simulink library "HORTISIM"  (R2021a)
settings: Solver=VariableStepAuto  StartTime=0.0  StopTime=10.0  RelTol=1e-3
undefined symbols (not defined in the file or in its folder): crop_params, heat_ic, heat_p, p_climate, params_fruit, scr_p, substrate_params, tp_tilapia, win_p, x0_climate, x0_crop, x0_fruit, x0_substrate, x0_tank_tilapia
libraries: $bdroot x10
(part 1 of 4)
settings Model: Creator=djoroya  LastModifiedBy=djoroya

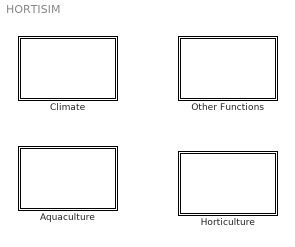
== system HORTISIM ==
  Aquaculture : Subsystem
  Climate : Subsystem
  Horticulture : Subsystem
  Other Functions : Subsystem

== system HORTISIM/Aquaculture ==
  Controls : Subsystem
  Models : Subsystem

== system HORTISIM/Climate ==
  Controls : Subsystem
  Models : Subsystem

== system HORTISIM/Horticulture ==
  Controls : Subsystem
  Models : Subsystem

== system HORTISIM/Other Functions ==
  Scalar2Bus Control Crop : Subsystem
  Scalar2Bus Control Climate : Subsystem
  Screen Connector : Subsystem
  Sec2Days : Gain  Gain=24*3600
  Temp2SatDensity : Subsystem
  Windows Connector : Subsystem
  Zero Element Screen : Subsystem
  Zero Element Windows : Subsystem
  cumfun : Subsystem
  parseExteriorClima : Subsystem
  sigmoi : Subsystem  mask{sigma=0}

== system HORTISIM/Aquaculture/Controls ==

== system HORTISIM/Aquaculture/Models ==
  Filter Species : Subsystem
      mask Display: image('$imagefile'); % Use "Edit Image" on toolstrip to change.
  Tank Model : Subsystem  mask{x0=x0_tank_tilapia, params=tp_tilapia}
      settings: PortSchema="{\"entries\":[{\"content\":{\"sides\":[{\"content\":{\"connectorIds\":[\"In1\",\"In2\"]},\"type\":\"ConnectorPlacement.EquallySpacedRectSide\",\"uuid\":\"0362ec3b-d1e8-482f-a4df-c7eb6405d3bb\"},{\"content\":{\"connectorIds\":[\"Out1\"],\"side\":\"RIGHT\"},\"type\":\"ConnectorPlacement.EquallySpacedRectSide\",\"uuid\":\"883d7bea-5680-4a36-94aa-1bdc656ec6e4\"},{\"content\":{\"connectorIds\":[\"In3\"],\"side\":\"TOP\"},\"type\":\"ConnectorPlacement.EquallySpacedRectSide\",\"uuid\":\"cb609290-e3df-4833-81b0-31186814fdae\"},{\"content\":{\"connectorIds\":[\"In4\",\"In5\"],\"side\":\"BOTTOM\"},\"type\":\"ConnectorPlacement.EquallySpacedRectSide\",\"uuid\":\"90a50527-453f-4e54-bcbc-22902a66f901\"}]},\"type\":\"ConnectorPlacement.EquallySpacedConnector\",\"uuid\":\"8e8832ba-26f8-49e0-87fc-105394dbe278\"}],\"packageUris\":[\"http://schema.mathworks.com/mf0/Connector/R2020b\"],\"version\":\"1.0\"}"
      mask Display: image('$imagefile'); % Use "Edit Image" on toolstrip to change.

== system HORTISIM/Climate/Controls ==
  CO2 Pump : Subsystem
      mask Display: image('$imagefile'); % Use "Edit Image" on toolstrip to change.
  Fogging Controler : Subsystem
      mask Display: image('$imagefile'); % Use "Edit Image" on toolstrip to change.
  Heating Controler : Subsystem  mask{params=heat_p, x0=heat_ic}
      mask Display: image('$imagefile'); % Use "Edit Image" on toolstrip to change.
  Screen Controler : Subsystem  mask{params=scr_p}
      mask Display: image('$imagefile'); % Use "Edit Image" on toolstrip to change.
  Windows Controler : Subsystem  mask{params=win_p}
      mask Display: image('$imagefile'); % Use "Edit Image" on toolstrip to change.

== system HORTISIM/Climate/Models ==
  Climate Model : Subsystem  mask{params=p_climate, x0=x0_climate}
      mask Display: image('$imagefile'); % Use "Edit Image" on toolstrip to change.

== system HORTISIM/Horticulture/Controls ==
  Ferrtirrigation Controler : Subsystem
      mask Display: image('$imagefile'); % Use "Edit Image" on toolstrip to change.
  Prune Policy : Subsystem
      mask Display: image('$imagefile'); % Use "Edit Image" on toolstrip to change.

== system HORTISIM/Horticulture/Models ==
  Crop Grow : Subsystem  mask{params=crop_params, x0=x0_crop}
      settings: PortSchema="{\"entries\":[{\"content\":{\"sides\":[{\"content\":{\"connectorIds\":[\"In1\"]},\"type\":\"ConnectorPlacement.EquallySpacedRectSide\",\"uuid\":\"7d52d4c6-bc72-40ae-ba7a-fef791f60555\"},{\"content\":{\"connectorIds\":[\"Out1\"],\"side\":\"RIGHT\"},\"type\":\"ConnectorPlacement.EquallySpacedRectSide\",\"uuid\":\"3a9c2840-361d-4677-a7cc-c5f954b33f07\"},{\"content\":{\"connectorIds\":[\"In2\",\"In3\"],\"side\":\"TOP\"},\"type\":\"ConnectorPlacement.EquallySpacedRectSide\",\"uuid\":\"4fc8b0ee-86a8-4f1e-9fcc-25f95949aa32\"},{\"content\":{\"connectorIds\":[],\"side\":\"BOTTOM\"},\"type\":\"ConnectorPlacement.EquallySpacedRectSide\",\"uuid\":\"254dc665-acaf-49d5-9184-a028de083de6\"}]},\"type\":\"ConnectorPlacement.EquallySpacedConnector\",\"uuid\":\"4a2a8912-594b-41a4-9c04-2b6ae0329b55\"}],\"packageUris\":[\"http://schema.mathworks.com/mf0/Connector/R2020b\"],\"version\":\"1.0\"}"
      mask Display: image('$imagefile'); % Use "Edit Image" on toolstrip to change.
  Fruit Partitioning1 : Subsystem  mask{x0=x0_fruit, params=params_fruit}
      mask Display: image('$imagefile'); % Use "Edit Image" on toolstrip to change.
  Substrate Bag : Subsystem  mask{x0=x0_substrate, params=substrate_params}
      mask Display: image('$imagefile'); % Use "Edit Image" on toolstrip to change.

== system HORTISIM/Other Functions/Scalar2Bus Control Crop ==
  Prune : Inport
  Harvest : Inport  Port=2
  Artificial Rad : Inport  Port=3
  Bus Creator : BusCreator  Inputs=3
  out : Outport
  wires:
  Prune/1 -> Bus Creator/1  "Prune"
  Harvest/1 -> Bus Creator/2  "Harvest"
  Artificial Rad/1 -> Bus Creator/3  "Artificial Rad"
  Bus Creator/1 -> out/1

== system HORTISIM/Other Functions/Scalar2Bus Control Climate ==
  Windows : Inport
  Screen : Inport  Port=2
  Fog : Inport  Port=3
  CO2 : Inport  Port=4
  Bus Creator : BusCreator  Inputs=4
  CoCl : Outport
  wires:
  Screen/1 -> Bus Creator/2  "Screen"
  Bus Creator/1 -> CoCl/1
  Windows/1 -> Bus Creator/1  "Windows"
  CO2/1 -> Bus Creator/4  "CO2"
  Fog/1 -> Bus Creator/3  "Fog"

== system HORTISIM/Other Functions/Screen Connector ==
  value : Inport
  gamma : Inport  Port=2
  beta : Inport  Port=3
  Bus Creator1 : BusCreator  Inputs=3
  out : Outport
  wires:
  beta/1 -> Bus Creator1/3  "beta"
  Bus Creator1/1 -> out/1
  value/1 -> Bus Creator1/1  "value"
  gamma/1 -> Bus Creator1/2  "gamma_max"

== system HORTISIM/Other Functions/Temp2SatDensity ==
  temp : Inport
  Constant1 : Constant  Value=4030
  Constant2 : Constant  Value=11.56
  Constant3 : Constant  Value=1.2978
  Divide : Product  Inputs=*/
  Exp : Math  SaturateOnIntegerOverflow=on
  Gain : Gain  Gain=-0.0046
  Minus : Sum  Inputs=+-
  Minus1 : Sum  Inputs=+-
  Product : Product
  Sum : Sum  Inputs=|++
  Zero ºC in Kelvin : Constant  Value=273.15
  sat rho : Outport
  wires:
  Zero ºC in Kelvin/1 -> Minus1/2
  Constant1/1 -> Divide/1
  temp/1 -> Minus1/1, Divide/2
  Divide/1 -> Minus/2
  Constant2/1 -> Minus/1
  Minus/1 -> Exp/1
  Minus1/1 -> Gain/1
  Gain/1 -> Sum/1
  Constant3/1 -> Sum/2
  Product/1 -> sat rho/1
  Exp/1 -> Product/1
  Sum/1 -> Product/2

== system HORTISIM/Other Functions/Windows Connector ==
  value : Inport
  AR : Inport  Port=2
  Bus Creator1 : BusCreator  Inputs=2
  out : Outport
  wires:
  Bus Creator1/1 -> out/1
  value/1 -> Bus Creator1/1  "value"
  AR/1 -> Bus Creator1/2  "AR"

== system HORTISIM/Other Functions/Zero Element Screen ==
  Bus Creator : BusCreator  Inputs=3
  Constant : Constant  Value=0
  Constant1 : Constant  Value=0
  beta : Constant  Value=0
  out : Outport
  wires:
  Bus Creator/1 -> out/1
  Constant/1 -> Bus Creator/1  "value"
  Constant1/1 -> Bus Creator/2  "gamma_max"
  beta/1 -> Bus Creator/3  "beta"

== system HORTISIM/Other Functions/Zero Element Windows ==
  Bus Creator : BusCreator  Inputs=2
  Constant : Constant  Value=0
  Constant1 : Constant  Value=0
  out : Outport
  wires:
  Bus Creator/1 -> out/1
  Constant/1 -> Bus Creator/1  "value"
  Constant1/1 -> Bus Creator/2  "AR"

== system HORTISIM/Other Functions/cumfun ==
  In1 : Inport
  If : If
  If Action Subsystem : Subsystem  TreatAsAtomicUnit=on
  Merge : Merge
  Subsystem : Subsystem
  Out1 : Outport
  wires:
  Subsystem/1(Out1) -> Merge/1
  In1/1 -> Subsystem/1(In1), If/1
  If/1 -> Subsystem/Action
  If/2 -> If Action Subsystem/Action
  If Action Subsystem/1(Out1) -> Merge/2
  Merge/1 -> Out1/1

== system HORTISIM/Other Functions/parseExteriorClima ==
  Array : Inport
  Bus Creator : BusCreator  Inputs=4
  Demux : Demux
  Bus : Outport
  wires:
  Bus Creator/1 -> Bus/1
  Demux/4 -> Bus Creator/4  "Wind"
  Array/1 -> Demux/1
  Demux/3 -> Bus Creator/3  "HR"
  Demux/1 -> Bus Creator/1  "Temp"
  Demux/2 -> Bus Creator/2  "Rad"

== system HORTISIM/Other Functions/sigmoi ==
  x : Inport
  Constant : Constant  Value=0.5
  Gain : Gain  Gain=sigma
  Gain1 : Gain  Gain=0.5
  Sum : Sum  Inputs=|++
  Tanh : Trigonometry  Operator=tanh
  y : Outport
  wires:
  x/1 -> Gain/1
  Gain/1 -> Tanh/1
  Tanh/1 -> Gain1/1
  Gain1/1 -> Sum/1
  Sum/1 -> y/1
  Constant/1 -> Sum/2

== system HORTISIM/Aquaculture/Models/Filter Species ==
  "Water " : Inport
  Bus Creator : BusCreator  Inputs=2
  Constant : Constant  Value=zeros(8,1)  VectorParams1D=off
  Constant1 : Constant
  State : Outport
  wires:
  Constant/1 -> Bus Creator/2  "R"
  Constant1/1 -> Bus Creator/1  "m"
  Bus Creator/1 -> State/1

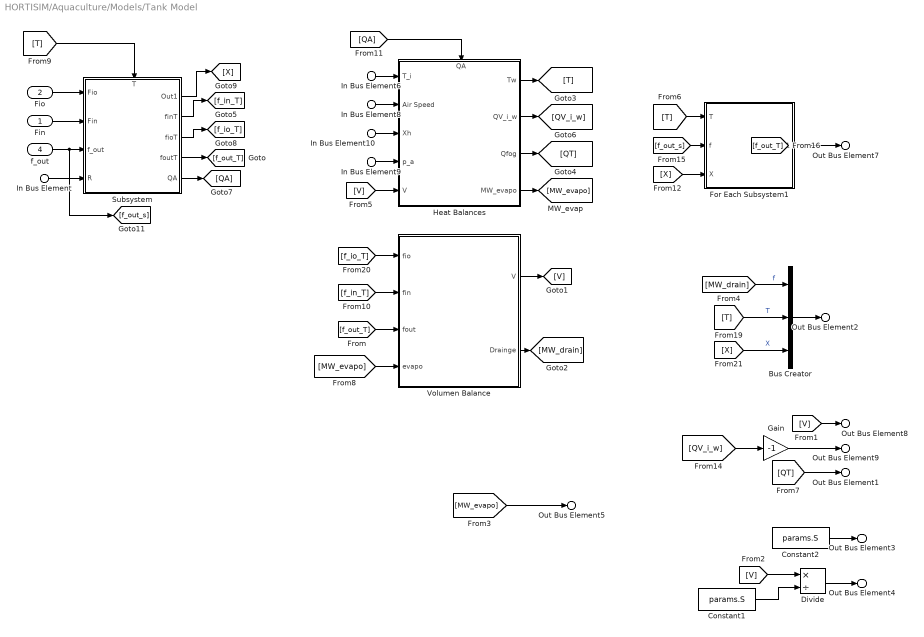
== system HORTISIM/Aquaculture/Models/Tank Model ==
  Fin : Inport
  Fio : Inport  Port=2
  In Bus Element6 : Inport  Port=3  PortName=Climate  Element=Temp.Tair
  In Bus Element8 : Inport  Port=3  PortName=Climate  Element=Gas.air_speed
  In Bus Element10 : Inport  Port=3  PortName=Climate  Element=Gas.Xh
  In Bus Element9 : Inport  Port=3  PortName=Climate  Element=Gas.p_a
  f_out : Inport  Port=4
  In Bus Element : Inport  Port=5  PortName=R  Element=R
  Bus Creator : BusCreator  Inputs=3  OutDataTypeStr=Bus: FLOW  NonVirtualBus=on
  Constant1 : Constant  Value=params.S
  Constant2 : Constant  Value=params.S
  Divide : Product  Inputs=*/
  For Each Subsystem1 : Subsystem  TreatAsAtomicUnit=on
  Gain : Gain  Gain=-1
  Heat Balances : Subsystem
      settings: PortSchema="{\"entries\":[{\"content\":{\"sides\":[{\"content\":{\"connectorIds\":[\"In1\",\"In2\",\"In3\",\"In4\",\"In5\"]},\"type\":\"ConnectorPlacement.EquallySpacedRectSide\",\"uuid\":\"26e11b66-a1c5-48e2-ab79-f5870a5f4091\"},{\"content\":{\"connectorIds\":[\"Out1\",\"Out2\",\"Out3\",\"Out4\"],\"side\":\"RIGHT\"},\"type\":\"ConnectorPlacement.EquallySpacedRectSide\",\"uuid\":\"91e62b2d-44c5-4f75-9dd0-4a25b0cbf311\"},{\"content\":{\"connectorIds\":[\"In6\"],\"side\":\"TOP\"},\"type\":\"ConnectorPlacement.EquallySpacedRectSide\",\"uuid\":\"31ab0e32-6ca6-469f-b51f-c6fe3cfb2917\"}]},\"type\":\"ConnectorPlacement.EquallySpacedConnector\",\"uuid\":\"d2f77916-79e9-406a-9ff1-65409dcf723a\"}],\"packageUris\":[\"http://schema.mathworks.com/mf0/Connector/R2020b\"],\"version\":\"1.0\"}"
  Subsystem : Subsystem
      settings: PortSchema="{\"entries\":[{\"content\":{\"sides\":[{\"content\":{\"connectorIds\":[\"In1\",\"In2\",\"In3\",\"In4\"]},\"type\":\"ConnectorPlacement.EquallySpacedRectSide\",\"uuid\":\"bf02c78f-575e-4f6b-a84d-6be35c02dacf\"},{\"content\":{\"connectorIds\":[\"Out1\",\"Out2\",\"Out3\",\"Out4\",\"Out5\"],\"side\":\"RIGHT\"},\"type\":\"ConnectorPlacement.EquallySpacedRectSide\",\"uuid\":\"62502bea-e4a7-4881-a7fa-104db083bc42\"},{\"content\":{\"connectorIds\":[\"In5\"],\"side\":\"TOP\"},\"type\":\"ConnectorPlacement.EquallySpacedRectSide\",\"uuid\":\"e34a6f62-efa4-430a-a08c-cf48cd0efcf5\"}]},\"type\":\"ConnectorPlacement.EquallySpacedConnector\",\"uuid\":\"9d683a7f-9e1c-4845-a964-e32ceb85a860\"}],\"packageUris\":[\"http://schema.mathworks.com/mf0/Connector/R2020b\"],\"version\":\"1.0\"}"
  Volumen Balance : Subsystem
  Out Bus Element7 : Outport  PortName=WaterTank  Element=Fout
  Out Bus Element8 : Outport  PortName=WaterTank  Element=V
  Out Bus Element9 : Outport  PortName=WaterTank  Element=QV
  Out Bus Element1 : Outport  PortName=WaterTank  Element=QT
  Out Bus Element2 : Outport  PortName=WaterTank  Element=Drainge
  Out Bus Element3 : Outport  PortName=WaterTank  Element=A_t
  Out Bus Element4 : Outport  PortName=WaterTank  Element=h
  Out Bus Element5 : Outport  PortName=WaterTank  Element=MW_QT
  wires:
  [QA] -> Heat Balances/6(QA)
  Subsystem/5(QA) -> [QA]
  [T] -> Subsystem/5(T)
  [MW_evapo] -> Out Bus Element5/1
  Constant1/1 -> Divide/2
  Divide/1 -> Out Bus Element4/1
  [V] -> Divide/1
  [V] -> Out Bus Element8/1
  [QT] -> Out Bus Element1/1
  Constant2/1 -> Out Bus Element3/1
  Gain/1 -> Out Bus Element9/1
  [QV_i_w] -> Gain/1
  In Bus Element6/1 -> Heat Balances/1(T_i)
  In Bus Element8/1 -> Heat Balances/2(Air Speed)
  In Bus Element10/1 -> Heat Balances/3(Xh)
  In Bus Element9/1 -> Heat Balances/4(p_a)
  Heat Balances/1(Tw) -> [T]
  Heat Balances/2(QV_i_w) -> [QV_i_w]
  Heat Balances/3(Qfog) -> [QT]
  Heat Balances/4(MW_evapo) -> [MW_evapo]
  [V] -> Heat Balances/5(V)
  [f_out_s] -> For Each Subsystem1/2(f)
  [X] -> For Each Subsystem1/3(X)
  [T] -> For Each Subsystem1/1(T)
  For Each Subsystem1/1(Out1) -> Out Bus Element7/1
  [MW_drain] -> Bus Creator/1  "f"
  [T] -> Bus Creator/2  "T"
  [X] -> Bus Creator/3  "X"
  Bus Creator/1 -> Out Bus Element2/1
  [f_io_T] -> Volumen Balance/1(fio)
  [f_in_T] -> Volumen Balance/2(fin)
  [f_out_T] -> Volumen Balance/3(fout)
  [MW_evapo] -> Volumen Balance/4(evapo)
  Volumen Balance/1(V) -> [V]
  Volumen Balance/2(Drainge) -> [MW_drain]
  Fio/1 -> Subsystem/1(Fio)
  Fin/1 -> Subsystem/2(Fin)
  In Bus Element/1 -> Subsystem/4(R)
  Subsystem/1(Out1) -> [X]
  Subsystem/2(finT) -> [f_in_T]
  Subsystem/3(fioT) -> [f_io_T]
  Subsystem/4(foutT) -> [f_out_T]
  f_out/1 -> [f_out_s], Subsystem/3(f_out)

== system HORTISIM/Climate/Controls/CO2 Pump ==
  hour : Inport
  MATLAB Function : MATLAB Function  TreatAsAtomicUnit=on
  MC_cc : Outport
  wires:
  MATLAB Function/1(MC_cc_i) -> MC_cc/1
  hour/1 -> MATLAB Function/1(hour)

== system HORTISIM/Climate/Controls/Fogging Controler ==
  HR : Inport
  HRMin : Inport  Port=2
  Bus Creator : BusCreator  Inputs=2
  Electric Model : Subsystem
  Subsystem : Subsystem
  Fog : Outport
  wires:
  Bus Creator/1 -> Fog/1
  Electric Model/1(Electrical Comsumption) -> Bus Creator/2  "Comsumptions"
  [Fog] -> Electric Model/1(Fog Motion), Bus Creator/1  "Signal"
  Subsystem/1(Fog Motion) -> [Fog]  "Fog"
  HR/1 -> Subsystem/1(HR)
  HRMin/1 -> Subsystem/2(HRMin)

== system HORTISIM/Climate/Controls/Heating Controler ==
  Tmax : Inport
  Tstart : Inport  Port=2
  In Bus Element : Inport  Port=3  PortName=EC  Element=Temp
  In Bus Element1 : Inport  Port=4  PortName=IC  Element=Temp.Tair
  Gain : Gain  Gain=params.power
  Integrator : Integrator  InitialCondition=x0.T  AbsoluteTolerance=0.001
  Sec2Days : Gain  Gain=24*3600
  Subsystem : Subsystem
  Subsystem2 : Subsystem
      settings: PortSchema="{\"entries\":[{\"content\":{\"sides\":[{\"content\":{\"connectorIds\":[\"In1\",\"In2\"]},\"type\":\"ConnectorPlacement.EquallySpacedRectSide\",\"uuid\":\"76a0539e-cd8b-47df-82d9-61971d3be914\"},{\"content\":{\"connectorIds\":[\"Out1\"],\"side\":\"RIGHT\"},\"type\":\"ConnectorPlacement.EquallySpacedRectSide\",\"uuid\":\"93f2ebb7-6ab4-4fcc-bc7a-3583f1db6e8e\"},{\"content\":{\"connectorIds\":[],\"side\":\"TOP\"},\"type\":\"ConnectorPlacement.EquallySpacedRectSide\",\"uuid\":\"b50a0ff6-3876-4dcb-8bb9-79340929aa80\"},{\"content\":{\"connectorIds\":[\"In3\"],\"side\":\"BOTTOM\"},\"type\":\"ConnectorPlacement.EquallySpacedRectSide\",\"uuid\":\"63f2a7a5-83ef-48e2-af90-7d61b47411e6\"}]},\"type\":\"ConnectorPlacement.EquallySpacedConnector\",\"uuid\":\"d97900b9-3143-4b55-b66d-f73dd0302926\"}],\"packageUris\":[\"http://schema.mathworks.com/mf0/Connector/R2020b\"],\"version\":\"1.0\"}"
  Heater : Outport  Unit=J
  Consumptions : Outport  Port=2
  State : Outport  Port=3
  wires:
  Integrator/1 -> Subsystem2/3(T), Subsystem/4(Th), State/1  "Th"
  Subsystem/2(dT_h_dt) -> Sec2Days/1
  Subsystem/1(QV_h_i) -> Heater/1  "QV_h_i"
  In Bus Element/1 -> Subsystem/3(T_e)
  In Bus Element1/1 -> Subsystem/1(T_i)
  Sec2Days/1 -> Integrator/1
  Subsystem2/1(y) -> Gain/1  "Control"
  Tmax/1 -> Subsystem2/2(Max)
  Tstart/1 -> Subsystem2/1(" Min")
  Gain/1 -> Subsystem/2(Q_h), Consumptions/1  "Q_h"

== system HORTISIM/Climate/Controls/Screen Controler ==
  In Bus Element : Inport  PortName=EC  Element=Rad
  Abs : Abs
  Bus Creator : BusCreator  Inputs=3
  Constant : Constant  Value=params.gamma_max
  Constant1 : Constant  Value=params.beta
  Gain : Gain  Gain=params.velocity
  Gain1 : Gain  Gain=params.Power
  Integrator : Integrator
  Minus : Sum  Inputs=+-
  Sec2Days : Gain  Gain=24*3600
  Subsystem : Subsystem
  Tanh : Trigonometry  Operator=tanh
  Screen : Outport
  " Consumptions" : Outport  Port=2
  wires:
  Constant1/1 -> Bus Creator/3  "beta"
  Constant/1 -> Bus Creator/1  "gamma_max"
  Bus Creator/1 -> Screen/1
  Abs/1 -> Gain1/1
  Gain/1 -> Sec2Days/1, Abs/1
  Subsystem/1(Out1) -> [Target]
  In Bus Element/1 -> Subsystem/1(In1)
  [Target] -> Minus/1
  Tanh/1 -> Gain/1
  Minus/1 -> Tanh/1
  Sec2Days/1 -> Integrator/1
  Integrator/1 -> Minus/2, Bus Creator/2  "value"
  Gain1/1 -> " Consumptions"/1  "Comsumptions"

== system HORTISIM/Climate/Controls/Windows Controler ==
  note: Subsystem1
  In Bus Element : Inport  PortName=IC  Element=QS.R_int
  In Bus Element1 : Inport  PortName=IC  Element=Temp.Tair
  In Bus Element2 : Inport  PortName=IC  Element=Gas.HRInt
  Tstart : Inport  Port=2
  Tmax : Inport  Port=3
  Hstart : Inport  Port=4
  Hmax : Inport  Port=5
  Abs : Abs  ZeroCross=off
  Bus Creator : BusCreator  Inputs=2
  Constant : Constant  Value=params.AR
  Gain : Gain  Gain=100/params.tau
  Gain1 : Gain  Gain=params.Power
  Integrator : Integrator
  Minus : Sum  Inputs=+-
  Sec2Days : Gain  Gain=24*3600
  Subsystem : Subsystem
      settings: PortSchema="{\"entries\":[{\"content\":{\"sides\":[{\"content\":{\"connectorIds\":[\"In1\",\"In2\",\"In3\",\"In4\",\"In5\",\"In6\"]},\"type\":\"ConnectorPlacement.EquallySpacedRectSide\",\"uuid\":\"18d05740-181f-409c-94ea-b42b6e57ea74\"},{\"content\":{\"connectorIds\":[\"Out1\"],\"side\":\"RIGHT\"},\"type\":\"ConnectorPlacement.EquallySpacedRectSide\",\"uuid\":\"978406c3-d241-44cd-a3e7-fe734e3a171e\"},{\"content\":{\"connectorIds\":[\"In7\"],\"side\":\"TOP\"},\"type\":\"ConnectorPlacement.EquallySpacedRectSide\",\"uuid\":\"b3c10a0e-c6d9-4444-97f2-9f0c7dea8ec9\"}]},\"type\":\"ConnectorPlacement.EquallySpacedConnector\",\"uuid\":\"429bf3f5-5806-495e-b66b-96810540e6d1\"}],\"packageUris\":[\"http://schema.mathworks.com/mf0/Connector/R2020b\"],\"version\":\"1.0\"}"
  Tanh : Trigonometry  Operator=tanh
  Windows : Outport
  Consumptions : Outport  Port=2
  wires:
  Constant/1 -> Bus Creator/2  "AR"
  Bus Creator/1 -> Windows/1
  Minus/1 -> Tanh/1
  Tanh/1 -> Gain/1
  Gain/1 -> Sec2Days/1, Abs/1
  Abs/1 -> Gain1/1
  Gain1/1 -> Consumptions/1  "Power"
  Sec2Days/1 -> Integrator/1
  Subsystem/1(y) -> Minus/1
  Hmax/1 -> Subsystem/6(HRMax)
  In Bus Element/1 -> Subsystem/7(Rad)
  Hstart/1 -> Subsystem/5(HRStart)
  In Bus Element2/1 -> Subsystem/4(HRInt)
  Integrator/1 -> Minus/2, Bus Creator/1  "value"
  Tmax/1 -> Subsystem/3(Tmax)
  In Bus Element1/1 -> Subsystem/2(Ti)
  Tstart/1 -> Subsystem/1(Tstart)

== system HORTISIM/Climate/Models/Climate Model ==
  In Bus Element14 : Inport  PortName=Ext  Element=QT
  In Bus Element1 : Inport  PortName=Ext  Element=QV
  In Bus Element2 : Inport  PortName=Ext  Element=CC
  In Bus Element7 : Inport  PortName=Ext  Element=A
  In Bus Element3 : Inport  Port=2  PortName=Control  Element=Fog
  In Bus Element5 : Inport  Port=2  PortName=Control  Element=Screen.gamma_max
  In Bus Element15 : Inport  Port=2  PortName=Control  Element=Screen.value
  In Bus Element16 : Inport  Port=2  PortName=Control  Element=Screen.beta
  In Bus Element6 : Inport  Port=2  PortName=Control  Element=CO2
  In Bus Element8 : Inport  Port=2  PortName=Control  Element=Windows.AR
  In Bus Element4 : Inport  Port=2  PortName=Control  Element=Windows.value
  In Bus Element9 : Inport  Port=3  PortName=EC  Element=HR
  In Bus Element10 : Inport  Port=3  PortName=EC  Element=Temp
  In Bus Element11 : Inport  Port=3  PortName=EC  Element=Temp
  In Bus Element12 : Inport  Port=3  PortName=EC  Element=Rad
  In Bus Element13 : Inport  Port=3  PortName=EC  Element=Wind
  Bus Creator : BusCreator  Inputs=3
  Bus Creator1 : BusCreator  Inputs=3
  Bus Creator2 : BusCreator  Inputs=2
  Bus Creator3 : BusCreator  Inputs=3
  Bus Creator4 : BusCreator  Inputs=2
  Gases Exchange : Subsystem
      settings: PortSchema="{\"entries\":[{\"content\":{\"sides\":[{\"content\":{\"connectorIds\":[\"In1\",\"In2\",\"In3\",\"In4\"]},\"type\":\"ConnectorPlacement.EquallySpacedRectSide\",\"uuid\":\"550da9a1-5f22-4db3-9ee3-e3750278f626\"},{\"content\":{\"connectorIds\":[\"Out1\"],\"side\":\"RIGHT\"},\"type\":\"ConnectorPlacement.EquallySpacedRectSide\",\"uuid\":\"cf559ec0-337d-42e7-96bb-a49ff9e682f6\"},{\"content\":{\"connectorIds\":[\"In5\"],\"side\":\"TOP\"},\"type\":\"ConnectorPlacement.EquallySpacedRectSide\",\"uuid\":\"d9874986-c35c-443c-9325-7a886074565b\"},{\"content\":{\"connectorIds\":[\"In6\",\"In7\"],\"side\":\"BOTTOM\"},\"type\":\"ConnectorPlacement.EquallySpacedRectSide\",\"uuid\":\"7f205c84-db2c-43a4-94ce-a6d2142a4e50\"}]},\"type\":\"ConnectorPlacement.EquallySpacedConnector\",\"uuid\":\"56c5cbc1-f580-43fc-9d79-62500ce9be4b\"}],\"packageUris\":[\"http://schema.mathworks.com/mf0/Connector/R2020b\"],\"version\":\"1.0\"}"
  Indoor Temperature Model : Subsystem
      settings: PortSchema="{\"entries\":[{\"content\":{\"sides\":[{\"content\":{\"connectorIds\":[\"In1\",\"In2\",\"In3\"]},\"type\":\"ConnectorPlacement.EquallySpacedRectSide\",\"uuid\":\"402556d7-b277-4cb3-8556-883bae99c69c\"},{\"content\":{\"connectorIds\":[\"Out1\",\"Out2\",\"Out3\",\"Out4\"],\"side\":\"RIGHT\"},\"type\":\"ConnectorPlacement.EquallySpacedRectSide\",\"uuid\":\"e8ec9f82-8759-4d98-a5e5-ef4db996ec8c\"},{\"content\":{\"connectorIds\":[\"In4\",\"In5\",\"In6\"],\"side\":\"TOP\"},\"type\":\"ConnectorPlacement.EquallySpacedRectSide\",\"uuid\":\"99d33cea-a089-4bcb-9505-68914c63f152\"},{\"content\":{\"connectorIds\":[\"Out5\"],\"side\":\"BOTTOM\"},\"type\":\"ConnectorPlacement.EquallySpacedRectSide\",\"uuid\":\"61ead6b3-0464-47f9-9f23-19f86056b325\"}]},\"type\":\"ConnectorPlacement.EquallySpacedConnector\",\"uuid\":\"a07dfd2f-7b40-4439-87f5-f093ac984b26\"}],\"packageUris\":[\"http://schema.mathworks.com/mf0/Connector/R2020b\"],\"version\":\"1.0\"}"
  Subsystem : Subsystem
      settings: PortSchema="{\"entries\":[{\"content\":{\"sides\":[{\"content\":{\"connectorIds\":[]},\"type\":\"ConnectorPlacement.EquallySpacedRectSide\",\"uuid\":\"35868875-f783-4ad4-af7a-8ba6d23e35d0\"},{\"content\":{\"connectorIds\":[\"Out1\"],\"side\":\"RIGHT\"},\"type\":\"ConnectorPlacement.EquallySpacedRectSide\",\"uuid\":\"2025d12d-e021-4399-bfe6-d7037c727539\"},{\"content\":{\"connectorIds\":[],\"side\":\"TOP\"},\"type\":\"ConnectorPlacement.EquallySpacedRectSide\",\"uuid\":\"3e424627-322e-4117-9014-21364a52cbdc\"},{\"content\":{\"connectorIds\":[\"In1\"],\"side\":\"BOTTOM\"},\"type\":\"ConnectorPlacement.EquallySpacedRectSide\",\"uuid\":\"db7a2526-7ee4-413d-8e1d-de852bb4cdfb\"}]},\"type\":\"ConnectorPlacement.EquallySpacedConnector\",\"uuid\":\"c6534136-4261-4144-9645-4fbbe9dd779a\"}],\"packageUris\":[\"http://schema.mathworks.com/mf0/Connector/R2020b\"],\"version\":\"1.0\"}"
  Out Bus Element : Outport  PortName=Climate  Element=Temp
  Out Bus Element1 : Outport  PortName=Climate  Element=QT
  Out Bus Element2 : Outport  PortName=Climate  Element=QS
  Out Bus Element3 : Outport  PortName=Climate  Element=Gas
  wires:
  In Bus Element16/1 -> Bus Creator3/3
  In Bus Element15/1 -> Bus Creator3/2
  In Bus Element5/1 -> Bus Creator3/1
  Bus Creator3/1 -> Indoor Temperature Model/5(Screen)
  Subsystem/1(Out1) -> Indoor Temperature Model/6(Gas)
  Bus Creator4/1 -> Indoor Temperature Model/1(Windows)
  In Bus Element8/1 -> Bus Creator4/1  "AR"
  In Bus Element4/1 -> Bus Creator4/2  "value"
  Gases Exchange/1(" Gas") -> Out Bus Element3/1, Subsystem/1(Gas)  "Gas"
  In Bus Element2/1 -> Gases Exchange/6(Carbon Consumption)
  Indoor Temperature Model/4(Condensation Heat) -> Gases Exchange/4(Condensation)
  Indoor Temperature Model/3(Ventilation Rate) -> Gases Exchange/3(Ventilation Rate)
  Indoor Temperature Model/1(Indoor Climate) -> Out Bus Element/1, Gases Exchange/1(Indoor Temperature)
  Indoor Temperature Model/2(Transpiration Heat) -> Gases Exchange/2(Transpiration Heat), Out Bus Element1/1
  Indoor Temperature Model/5(Solar Energy) -> Out Bus Element2/1
  In Bus Element3/1 -> Indoor Temperature Model/4(Fog)
  In Bus Element6/1 -> Gases Exchange/7(CO2 Pump)
  In Bus Element12/1 -> Bus Creator1/2
  In Bus Element13/1 -> Bus Creator1/3
  In Bus Element11/1 -> Bus Creator1/1
  Bus Creator1/1 -> Indoor Temperature Model/2(EC)
  Bus Creator2/1 -> Gases Exchange/5(EC)
  In Bus Element9/1 -> Bus Creator2/1
  In Bus Element10/1 -> Bus Creator2/2
  In Bus Element1/1 -> Bus Creator/2
  In Bus Element14/1 -> Bus Creator/1
  Bus Creator/1 -> Indoor Temperature Model/3(External)
  In Bus Element7/1 -> Bus Creator/3

== system HORTISIM/Horticulture/Controls/Ferrtirrigation Controler ==
  note: $kg\{H_2O\}/(s\cdot plant)$
  Bus Creator : BusCreator  Inputs=3  OutDataTypeStr=Bus: FLOW  NonVirtualBus=on
  Irrigation Controler : Subsystem
  "[Kelvin]" : Constant  Value=273.15 + 10
  kg/m^3 : Constant  Value=0.1 +zeros(8,1)
  Irrigation : Outport
  wires:
  Bus Creator/1 -> Irrigation/1
  "[Kelvin]"/1 -> Bus Creator/2  "T"
  Irrigation Controler/1(Irrigation) -> Bus Creator/1  "f"
  kg/m^3/1 -> Bus Creator/3  "X"

== system HORTISIM/Horticulture/Controls/Prune Policy ==
  Crop : Inport
  Bus Selector : BusSelector  OutputSignals=LAI
  Constant : Constant  Value=5
  Constant1 : Constant  Value=0
  Gain : Gain  Gain=0.01/(3600*24)
  Min : MinMax  Function=max  Inputs=2  ZeroCross=off
  Minus : Sum  Inputs=-+
  Prune : Outport
  wires:
  Constant/1 -> Minus/1
  Minus/1 -> Gain/1
  Gain/1 -> Min/1
  Constant1/1 -> Min/2
  Min/1 -> Prune/1
  Crop/1 -> Bus Selector/1
  Bus Selector/1 -> Minus/2  "<LAI>"

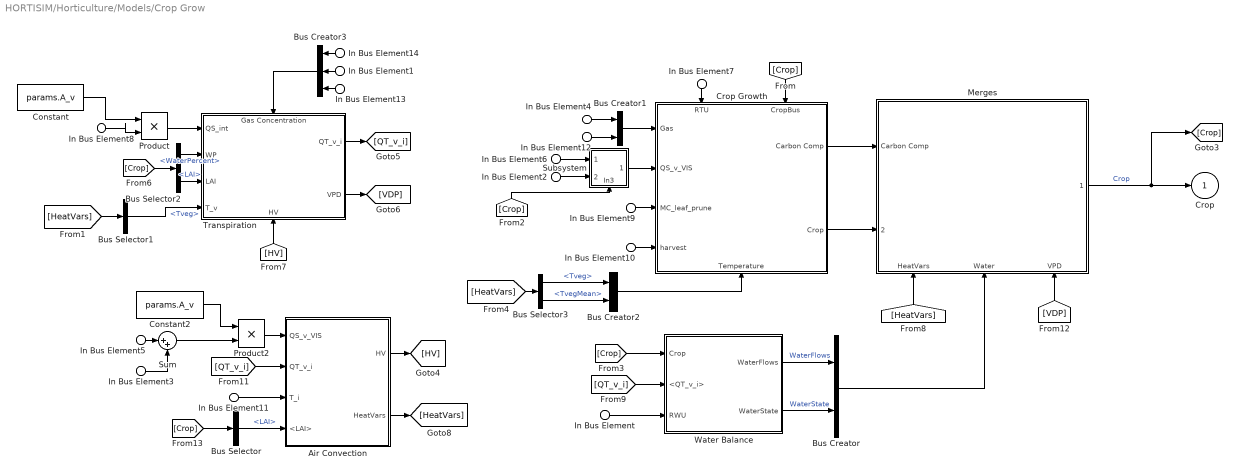
== system HORTISIM/Horticulture/Models/Crop Grow ==
  In Bus Element8 : Inport  PortName=Climate  Element=QS.R_int
  In Bus Element3 : Inport  PortName=Climate  Element=QS.R_int
  In Bus Element2 : Inport  PortName=Climate  Element=QS.R_int
  In Bus Element11 : Inport  PortName=Climate  Element=Temp.Tair
  In Bus Element4 : Inport  PortName=Climate  Element=Gas.C_c
  In Bus Element12 : Inport  PortName=Climate  Element=Gas.rho_i
  In Bus Element13 : Inport  PortName=Climate  Element=Gas.rho_i
  In Bus Element1 : Inport  PortName=Climate  Element=Gas.C_c_ppm
  In Bus Element14 : Inport  PortName=Climate  Element=Gas.C_w
  In Bus Element9 : Inport  Port=2  PortName=Control  Element=Prune
  In Bus Element5 : Inport  Port=2  PortName=Control  Element=Artificial Rad
  In Bus Element6 : Inport  Port=2  PortName=Control  Element=Artificial Rad
  In Bus Element10 : Inport  Port=2  PortName=Control  Element=Harvest
  In Bus Element : Inport  Port=3  PortName=Substrate  Element=Uptake.Water
  In Bus Element7 : Inport  Port=3  PortName=Substrate  Element=Uptake.Nutrients
  Air Convection : Subsystem
  Bus Creator : BusCreator  Inputs=2
  Bus Creator1 : BusCreator  Inputs=2
  Bus Creator2 : BusCreator  Inputs=2
  Bus Creator3 : BusCreator  Inputs=3
  Bus Selector : BusSelector  OutputSignals=LAI
  Bus Selector1 : BusSelector  OutputSignals=Tveg
  Bus Selector2 : BusSelector  OutputSignals=WaterPercent,LAI
  Bus Selector3 : BusSelector  OutputSignals=Tveg,TvegMean
  Constant : Constant  Value=params.A_v
  Constant2 : Constant  Value=params.A_v
  Crop Growth : Subsystem
      settings: PortSchema="{\"entries\":[{\"content\":{\"sides\":[{\"content\":{\"connectorIds\":[\"In1\",\"In2\",\"In3\",\"In4\"]},\"type\":\"ConnectorPlacement.EquallySpacedRectSide\",\"uuid\":\"e694206d-cf53-43ea-b790-8b83ac78aa3a\"},{\"content\":{\"connectorIds\":[\"Out1\",\"Out2\"],\"side\":\"RIGHT\"},\"type\":\"ConnectorPlacement.EquallySpacedRectSide\",\"uuid\":\"93817abb-865a-4529-a53b-9aa59cd1156c\"},{\"content\":{\"connectorIds\":[\"In5\",\"In6\"],\"side\":\"TOP\"},\"type\":\"ConnectorPlacement.EquallySpacedRectSide\",\"uuid\":\"edd59083-b991-4826-870e-7da3bc3e48d4\"},{\"content\":{\"connectorIds\":[\"In7\"],\"side\":\"BOTTOM\"},\"type\":\"ConnectorPlacement.EquallySpacedRectSide\",\"uuid\":\"aa2b3153-bf16-47ed-b19e-45b92f713263\"}]},\"type\":\"ConnectorPlacement.EquallySpacedConnector\",\"uuid\":\"72640b1e-82d8-4725-bb34-7435bfc9f969\"}],\"packageUris\":[\"http://schema.mathworks.com/mf0/Connector/R2020b\"],\"version\":\"1.0\"}"
  Merges : Subsystem
      settings: PortSchema="{\"entries\":[{\"content\":{\"sides\":[{\"content\":{\"connectorIds\":[\"In1\",\"In2\"]},\"type\":\"ConnectorPlacement.EquallySpacedRectSide\",\"uuid\":\"f4887da6-2928-4f39-8f5f-a84d343119b4\"},{\"content\":{\"connectorIds\":[\"Out1\"],\"side\":\"RIGHT\"},\"type\":\"ConnectorPlacement.EquallySpacedRectSide\",\"uuid\":\"0df0d8c4-f19c-45da-a42d-26f0e872c274\"},{\"content\":{\"connectorIds\":[],\"side\":\"TOP\"},\"type\":\"ConnectorPlacement.EquallySpacedRectSide\",\"uuid\":\"3b0cc3f6-1cfb-43ac-8908-74a7a76931e3\"},{\"content\":{\"connectorIds\":[\"In3\",\"In4\",\"In5\"],\"side\":\"BOTTOM\"},\"type\":\"ConnectorPlacement.EquallySpacedRectSide\",\"uuid\":\"7e6672ca-68aa-4c3f-955a-240d8575a2c6\"}]},\"type\":\"ConnectorPlacement.EquallySpacedConnector\",\"uuid\":\"a8299565-1b25-4490-849f-a8fa281592c1\"}],\"packageUris\":[\"http://schema.mathworks.com/mf0/Connector/R2020b\"],\"version\":\"1.0\"}"
  Product : Product
  Product2 : Product
  Subsystem : Subsystem
      settings: PortSchema="{\"entries\":[{\"content\":{\"sides\":[{\"content\":{\"connectorIds\":[\"In1\",\"In2\"]},\"type\":\"ConnectorPlacement.EquallySpacedRectSide\",\"uuid\":\"c9e251e2-f19d-4856-b15c-3b9f1eb64f83\"},{\"content\":{\"connectorIds\":[\"Out1\"],\"side\":\"RIGHT\"},\"type\":\"ConnectorPlacement.EquallySpacedRectSide\",\"uuid\":\"10734817-c937-42fb-8ae5-9505620c6f0f\"},{\"content\":{\"connectorIds\":[],\"side\":\"TOP\"},\"type\":\"ConnectorPlacement.EquallySpacedRectSide\",\"uuid\":\"8c056440-d8bf-4ff4-85aa-0f6a5eb7f23f\"},{\"content\":{\"connectorIds\":[\"In3\"],\"side\":\"BOTTOM\"},\"type\":\"ConnectorPlacement.EquallySpacedRectSide\",\"uuid\":\"dd07dcd8-5298-4126-bdbb-0b047f66f0f4\"}]},\"type\":\"ConnectorPlacement.EquallySpacedConnector\",\"uuid\":\"13e72cfa-9d8f-4756-adac-f24fb0238c2a\"}],\"packageUris\":[\"http://schema.mathworks.com/mf0/Connector/R2020b\"],\"version\":\"1.0\"}"
  Sum : Sum  Inputs=|++
  Transpiration : Subsystem
      settings: PortSchema="{\"entries\":[{\"content\":{\"sides\":[{\"content\":{\"connectorIds\":[\"In1\",\"In2\",\"In3\",\"In4\"]},\"type\":\"ConnectorPlacement.EquallySpacedRectSide\",\"uuid\":\"d6bbd0cc-329a-44d5-b58b-a93078f7e5d1\"},{\"content\":{\"connectorIds\":[\"Out1\",\"Out2\"],\"side\":\"RIGHT\"},\"type\":\"ConnectorPlacement.EquallySpacedRectSide\",\"uuid\":\"249abf44-6c9b-4b00-a2f9-2043ee582e13\"},{\"content\":{\"connectorIds\":[\"In5\"],\"side\":\"TOP\"},\"type\":\"ConnectorPlacement.EquallySpacedRectSide\",\"uuid\":\"efa2d349-63e9-4701-9d30-a0c2adbee945\"},{\"content\":{\"connectorIds\":[\"In6\"],\"side\":\"BOTTOM\"},\"type\":\"ConnectorPlacement.EquallySpacedRectSide\",\"uuid\":\"decf1794-1744-434d-adf6-c7060d48f04b\"}]},\"type\":\"ConnectorPlacement.EquallySpacedConnector\",\"uuid\":\"1e3e15aa-c080-4684-9da5-24f03928e17f\"}],\"packageUris\":[\"http://schema.mathworks.com/mf0/Connector/R2020b\"],\"version\":\"1.0\"}"
  Water Balance : Subsystem
  Crop : Outport
  wires:
  Merges/1("    ") -> Crop/1, [Crop]  "Crop"
  In Bus Element4/1 -> Bus Creator1/1
  In Bus Element12/1 -> Bus Creator1/2
  Bus Selector3/2 -> Bus Creator2/2  "<TvegMean>"
  [HV] -> Transpiration/6(HV)
  Bus Creator3/1 -> Transpiration/5(Gas Concentration)
  Bus Selector2/1 -> Transpiration/2(WP)  "<WaterPercent>"
  [Crop] -> Bus Selector2/1
  Bus Selector2/2 -> Transpiration/3(LAI)  "<LAI>"
  Transpiration/1(QT_v_i) -> [QT_v_i]
  Transpiration/2(VPD) -> [VDP]
  [VDP] -> Merges/5(VPD)
  [Crop] -> Bus Selector/1
  Bus Selector1/1 -> Transpiration/4(T_v)  "<Tveg>"
  [HeatVars] -> Merges/3(HeatVars)
  Bus Creator1/1 -> Crop Growth/1(Gas)
  In Bus Element9/1 -> Crop Growth/3(MC_leaf_prune)
  Bus Creator2/1 -> Crop Growth/7(Temperature)
  Crop Growth/1("Carbon Comp   ") -> Merges/1("Carbon Comp   ")
  Crop Growth/2(Crop) -> Merges/2(" ")
  [Crop] -> Water Balance/1(Crop)
  [QT_v_i] -> Water Balance/2(<QT_v_i>)
  [QT_v_i] -> Air Convection/2(QT_v_i)
  In Bus Element11/1 -> Air Convection/3(T_i)
  Bus Selector/1 -> Air Convection/4(<LAI>)  "<LAI>"
  Air Convection/1(HV) -> [HV]
  Air Convection/2(HeatVars) -> [HeatVars]
  [Crop] -> Crop Growth/6(CropBus)
  In Bus Element14/1 -> Bus Creator3/1
  In Bus Element1/1 -> Bus Creator3/2
  In Bus Element13/1 -> Bus Creator3/3
  Constant/1 -> Product/1
  In Bus Element8/1 -> Product/2
  Product/1 -> Transpiration/1(QS_int)
  Product2/1 -> Air Convection/1(QS_v_VIS)
  Constant2/1 -> Product2/1
  In Bus Element5/1 -> Sum/1
  In Bus Element3/1 -> Sum/2
  Sum/1 -> Product2/2
  In Bus Element6/1 -> Subsystem/1(In1)
  In Bus Element2/1 -> Subsystem/2(In2)
  Subsystem/1(Out1) -> Crop Growth/2(QS_v_VIS)
  In Bus Element7/1 -> Crop Growth/5(RTU)
  Water Balance/1(WaterFlows) -> Bus Creator/1  "WaterFlows"
  Water Balance/2(WaterState) -> Bus Creator/2  "WaterState"
  Bus Creator/1 -> Merges/4(Water)
  [HeatVars] -> Bus Selector1/1
  [HeatVars] -> Bus Selector3/1
  Bus Selector3/1 -> Bus Creator2/1  "<Tveg>"
  In Bus Element/1 -> Water Balance/3(RWU)
  In Bus Element10/1 -> Crop Growth/4(harvest)
  [Crop] -> Subsystem/3(In3)

== system HORTISIM/Horticulture/Models/Fruit Partitioning1 ==
  In Bus Element : Inport  PortName=Crop  Element=Tsum
  In Bus Element1 : Inport  PortName=Crop  Element=HeatVars.TvegMean
  In Bus Element3 : Inport  PortName=Crop  Element=plants_density
  In Bus Element4 : Inport  PortName=Crop  Element=Carbon.Cfruit
  Integrator : Integrator  InitialCondition=1e-3
  MATLAB Function : MATLAB Function  TreatAsAtomicUnit=on
  Scope : Scope  NumInputPorts=2
  Scope1 : Scope
  Fruit Distribution : Outport
  wires:
  In Bus Element4/1 -> Scope/1, MATLAB Function/1(Cfruit)
  In Bus Element/1 -> MATLAB Function/2(Tsum)
  MATLAB Function/1(dCmdt) -> Integrator/1
  Integrator/1 -> MATLAB Function/3(Cfruit_mature), Fruit Distribution/1, Scope/2
  In Bus Element1/1 -> MATLAB Function/4(T)
  MATLAB Function/2(DT) -> Scope1/1

== system HORTISIM/Horticulture/Models/Substrate Bag ==
  note: $kg\{H_2O\}/m^2$
  note: $kg\{H_2O\}/(s\cdot m^2)$
  note: $kg\{H_2O\}/(s\cdot m^2)$
  note: $kg\{H_2O\}/(s\cdot m^2)$
  Crop : Inport
  Irrigation : Inport  Port=2
  Bus Creator : BusCreator  Inputs=3
  Bus Creator1 : BusCreator  Inputs=2
  Bus Creator2 : BusCreator  Inputs=4
  Bus Selector : BusSelector  OutputSignals=Nutrients.Demand,Water.WaterFlows.WaterDemand
  Bus Selector1 : BusSelector  OutputSignals=f
  Nutrient Balance : Subsystem
      settings: PortSchema="{\"entries\":[{\"content\":{\"sides\":[{\"content\":{\"connectorIds\":[\"In1\",\"In2\"]},\"type\":\"ConnectorPlacement.EquallySpacedRectSide\",\"uuid\":\"1a00bf92-a9c2-4ff2-a957-dcbceaefca92\"},{\"content\":{\"connectorIds\":[\"Out1\",\"Out2\",\"Out3\"],\"side\":\"RIGHT\"},\"type\":\"ConnectorPlacement.EquallySpacedRectSide\",\"uuid\":\"e56bd997-d011-4238-be11-f6e3de25f00c\"},{\"content\":{\"connectorIds\":[\"In3\"],\"side\":\"TOP\"},\"type\":\"ConnectorPlacement.EquallySpacedRectSide\",\"uuid\":\"b2f1d1bf-662b-4d11-ab71-7a2cc6ac889e\"}]},\"type\":\"ConnectorPlacement.EquallySpacedConnector\",\"uuid\":\"f2308665-0f29-4c83-a9f8-08128e360e13\"}],\"packageUris\":[\"http://schema.mathworks.com/mf0/Connector/R2020b\"],\"version\":\"1.0\"}"
  Subsystem3 : Subsystem
  State : Outport
  wires:
  Irrigation/1 -> Nutrient Balance/1(Irrigation), Bus Selector1/1
  Bus Selector1/1 -> Subsystem3/2(Irrigation)  "<f>"
  Crop/1 -> Bus Selector/1
  Subsystem3/2(C_ws) -> Bus Creator2/1, Bus Creator/2  "SusWater"
  Subsystem3/3(f_drainge) -> Bus Creator/3  "drainge"
  Bus Creator1/1 -> Bus Creator2/4  "Uptake"
  Subsystem3/1(WaterUptake) -> Bus Creator1/1, Bus Creator/1  "Water"
  Nutrient Balance/3(RealNutrientUptake) -> Bus Creator1/2  "Nutrients"
  Bus Selector/2 -> Subsystem3/1(Demand)  "<WaterDemand>"
  Bus Creator2/1 -> State/1
  Bus Creator/1 -> [W]
  [W] -> Nutrient Balance/3(Water)
  Nutrient Balance/1(Drainge) -> [Drain]  "Drainge"
  [Drain] -> Bus Creator2/2  "Drainge"
  Nutrient Balance/2(Mass In Sustrate) -> [Mass]  "MassX"
  [Mass] -> Bus Creator2/3  "Mass"
  Bus Selector/1 -> [NutrientDemand]  "<Demand>"
  [NutrientDemand] -> Nutrient Balance/2(NutrientDemand)

== system HORTISIM/Other Functions/cumfun/If Action Subsystem ==
  Action Port : ActionPort  ActionPortLabel=else
  Constant : Constant  Value=0
  Out1 : Outport
  wires:
  Constant/1 -> Out1/1

== system HORTISIM/Other Functions/cumfun/Subsystem ==
  In1 : Inport
  Action Port : ActionPort  ActionPortLabel=if(u1 > 0)
  Constant : Constant
  Constant1 : Constant  Value=3
  Exp : Math  SaturateOnIntegerOverflow=on
  Gain : Gain  Gain=-1
  Minus : Sum  Inputs=+-
  Square : Math  Operator=pow  SaturateOnIntegerOverflow=on
  Out1 : Outport
  wires:
  In1/1 -> Gain/1
  Minus/1 -> Out1/1
  Constant/1 -> Minus/1
  Gain/1 -> Square/1
  Constant1/1 -> Square/2
  Square/1 -> Exp/1
  Exp/1 -> Minus/2

== system HORTISIM/Aquaculture/Models/Tank Model/For Each Subsystem1 ==
  T : Inport
  f : Inport  Port=2  Partition=on  PartitionDimension=1  PartitionWidth=1  PartitionOffset=0
  X : Inport  Port=3
  Bus Creator : BusCreator  Inputs=3  OutDataTypeStr=Bus: FLOW  NonVirtualBus=on
  For Each : ForEach  DisableCoverage=on
  Out1 : Outport  ConcatenationDimension=1
  wires:
  T/1 -> Bus Creator/2  "T"
  f/1 -> Bus Creator/1  "f"
  X/1 -> Bus Creator/3  "X"
  Bus Creator/1 -> Out1/1

== system HORTISIM/Aquaculture/Models/Tank Model/Heat Balances ==
  T_i : Inport
  Air Speed : Inport  Port=2
  Xh : Inport  Port=3
  p_a : Inport  Port=4
  V : Inport  Port=5
  QA : Inport  Port=6
  Constant1 : Constant  Value=params.S
  Constant3 : Constant  Value=params.S
  Constant4 : Constant  Value=1.5
  Constant5 : Constant  Value=1.5
  Constant6 : Constant  Value=params.Twall
  Convection Air 2 Water Tanl Surface : Subsystem
  Convection Air 2 Water Tanl Surface1 : Subsystem
  Energy Balance : Subsystem
      settings: PortSchema="{\"entries\":[{\"content\":{\"sides\":[{\"content\":{\"connectorIds\":[\"In1\",\"In2\"]},\"type\":\"ConnectorPlacement.EquallySpacedRectSide\",\"uuid\":\"351dfee1-09c7-4321-9b33-423602220319\"},{\"content\":{\"connectorIds\":[\"Out1\"],\"side\":\"RIGHT\"},\"type\":\"ConnectorPlacement.EquallySpacedRectSide\",\"uuid\":\"92d6c083-190c-455c-8aef-b1925742528e\"},{\"content\":{\"connectorIds\":[\"In3\",\"In4\"],\"side\":\"TOP\"},\"type\":\"ConnectorPlacement.EquallySpacedRectSide\",\"uuid\":\"d8c819af-ff3d-42e7-8edd-277d07e80549\"},{\"content\":{\"connectorIds\":[\"In5\"],\"side\":\"BOTTOM\"},\"type\":\"ConnectorPlacement.EquallySpacedRectSide\",\"uuid\":\"a5e7f711-a00c-4a78-8adb-572186bb4217\"}]},\"type\":\"ConnectorPlacement.EquallySpacedConnector\",\"uuid\":\"109a8411-c568-42b4-8b05-82c996bc6781\"}],\"packageUris\":[\"http://schema.mathworks.com/mf0/Connector/R2020b\"],\"version\":\"1.0\"}"
  Gain1 : Gain  Gain=params.wall_gain
  Transpiration : Subsystem
  Tw : Outport
  QV_i_w : Outport  Port=2
  Qfog : Outport  Port=3
  MW_evapo : Outport  Port=4
  wires:
  QA/1 -> Energy Balance/3(QA)
  T_i/1 -> Convection Air 2 Water Tanl Surface/1(T_i)
  V/1 -> Energy Balance/2(V)
  Constant5/1 -> Convection Air 2 Water Tanl Surface1/4(d_t)
  Gain1/1 -> Energy Balance/5(QV_wall_water)  "QV_wall_water"
  Transpiration/1(QT) -> Energy Balance/4(QT), Qfog/1  "QT"
  Xh/1 -> Transpiration/2(Xh)
  Constant6/1 -> Convection Air 2 Water Tanl Surface1/3(T_wall)
  Energy Balance/1(Out1) -> [Tw], Tw/1
  Constant1/1 -> Convection Air 2 Water Tanl Surface1/2(A_t)
  Constant4/1 -> Convection Air 2 Water Tanl Surface/4(d_t)
  Transpiration/2(Evaporation) -> MW_evapo/1
  Convection Air 2 Water Tanl Surface1/1(QV_i_w) -> Gain1/1
  Constant3/1 -> Convection Air 2 Water Tanl Surface/2(A_t)
  Convection Air 2 Water Tanl Surface/1(QV_i_w) -> Energy Balance/1(QV_i_W), QV_i_w/1  "QV_i_W"
  [Tw] -> Transpiration/3(Tw)
  p_a/1 -> Transpiration/4(p_a)
  [Tw] -> Convection Air 2 Water Tanl Surface/3(T_w)
  [Tw] -> Convection Air 2 Water Tanl Surface1/1(T_w)
  Air Speed/1 -> [air_speed]
  [air_speed] -> Transpiration/1(Air Speed)
  [air_speed] -> Convection Air 2 Water Tanl Surface/5(wind_speed)

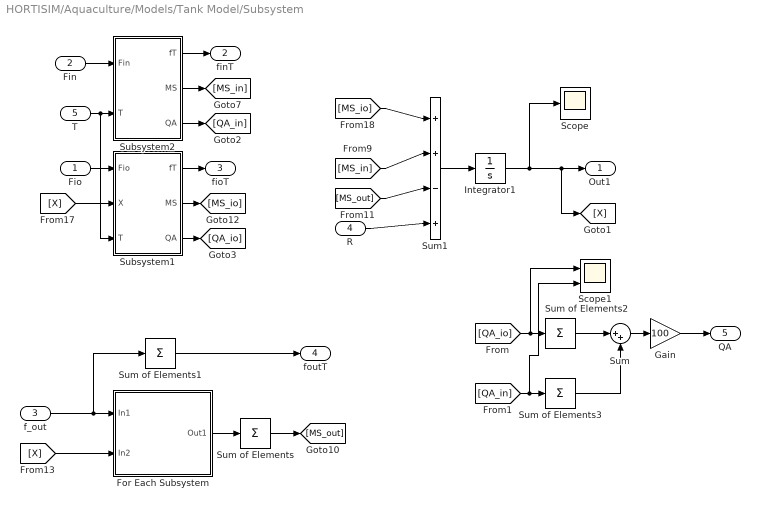
== system HORTISIM/Aquaculture/Models/Tank Model/Subsystem ==
  Fio : Inport
  Fin : Inport  Port=2
  f_out : Inport  Port=3
  R : Inport  Port=4
  T : Inport  Port=5
  For Each Subsystem : Subsystem  TreatAsAtomicUnit=on
  Gain : Gain  Gain=100
  Integrator1 : Integrator  InitialCondition=x0.X
  Scope : Scope
  Scope1 : Scope  NumInputPorts=2
  Subsystem1 : Subsystem
  Subsystem2 : Subsystem
  Sum : Sum  Inputs=|++
  Sum of Elements : Sum  Inputs=+  CollapseMode=Specified dimension  CollapseDim=2
  Sum of Elements1 : Sum  Inputs=+  CollapseDim=2
  Sum of Elements2 : Sum  Inputs=+
  Sum of Elements3 : Sum  Inputs=+
  Sum1 : Sum  Inputs=+|+-+
  Out1 : Outport
  finT : Outport  Port=2
  fioT : Outport  Port=3
  foutT : Outport  Port=4
  QA : Outport  Port=5
  wires:
  Sum/1 -> Gain/1
  Gain/1 -> QA/1
  Sum of Elements3/1 -> Sum/2
  Sum of Elements2/1 -> Sum/1
  [QA_in] -> Sum of Elements3/1, Scope1/2
  [QA_io] -> Sum of Elements2/1, Scope1/1
  Subsystem1/3(QA) -> [QA_io]
  Subsystem2/3(QA) -> [QA_in]
  T/1 -> Subsystem2/2(T), Subsystem1/3(T)
  R/1 -> Sum1/4
  [X] -> Subsystem1/2(X)
  Fio/1 -> Subsystem1/1(Fio)
  Subsystem1/2(MS) -> [MS_io]
  [MS_out] -> Sum1/3
  [MS_io] -> Sum1/1
  Sum of Elements/1 -> [MS_out]
  [MS_in] -> Sum1/2
  f_out/1 -> Sum of Elements1/1, For Each Subsystem/1(In1)
  Subsystem2/2(MS) -> [MS_in]
  Integrator1/1 -> [X], Out1/1, Scope/1
  Sum of Elements1/1 -> foutT/1
  For Each Subsystem/1(Out1) -> Sum of Elements/1
  Fin/1 -> Subsystem2/1(Fin)
  Sum1/1 -> Integrator1/1
  Subsystem1/1(fT) -> fioT/1
  [X] -> For Each Subsystem/2(In2)
  Subsystem2/1(fT) -> finT/1

== system HORTISIM/Aquaculture/Models/Tank Model/Volumen Balance ==
  fio : Inport
  fin : Inport  Port=2
  fout : Inport  Port=3
  evapo : Inport  Port=4
  Constant : Constant  Value=params.h_max * params.S
  Integrator : Integrator  InitialCondition=params.S * x0.h
  Minus : Sum  Inputs=+-
  Scope : Scope  NumInputPorts=2
  Sum : Sum  Inputs=+|+---
  cumfun : $bdroot/Other  Functions/cumfun  SystemSampleTime=-1  VariantActivationTime=update diagram  Latency=0  AutoFrameSizeCalculation=off
  seconds to days : Gain  Gain=(3600*24)
  V : Outport
  Drainge : Outport  Port=2
  wires:
  seconds to days/1 -> Integrator/1
  cumfun/1 -> Drainge/1, [MW_drain_max], Scope/1
  Integrator/1 -> Minus/1, V/1, Scope/2
  [MW_drain_max] -> Sum/4
  Sum/1 -> seconds to days/1
  fout/1 -> Sum/3
  evapo/1 -> Sum/5
  Minus/1 -> cumfun/1
  Constant/1 -> Minus/2
  fio/1 -> Sum/1
  fin/1 -> Sum/2

== system HORTISIM/Climate/Controls/Fogging Controler/Electric Model ==
  Fog Motion : Inport
  Derivative : Derivative
  Scope : Scope
  Electrical Comsumption : Outport
  wires:
  Fog Motion/1 -> Derivative/1
  Derivative/1 -> Scope/1, Electrical Comsumption/1

== system HORTISIM/Climate/Controls/Fogging Controler/Subsystem ==
  HR : Inport
  HRMin : Inport  Port=2
  Constant : Constant  Value=60
  Gain : Gain  Gain=0
  Subsystem2 : Subsystem
  Fog Motion : Outport
  wires:
  HR/1 -> Subsystem2/1(Signal)
  HRMin/1 -> Subsystem2/2(" Min")
  Constant/1 -> Subsystem2/3(Max)
  Subsystem2/1(y) -> Gain/1
  Gain/1 -> Fog Motion/1

== system HORTISIM/Climate/Controls/Heating Controler/Subsystem ==
  T_i : Inport
  Q_h : Inport  Port=2
  T_e : Inport  Port=3
  Th : Inport  Port=4
  Constant : Constant  Value=params.A_i
  Constant1 : Constant  Value=params.c
  Constant2 : Constant  Value=params.A_e
  Product : Product
  Subsystem1 : Subsystem
  Subsystem2 : Subsystem
  Sum : Sum  Inputs=|-+-
  QV_h_i : Outport
  dT_h_dt : Outport  Port=2
  wires:
  Constant2/1 -> Subsystem2/2(A_h_exp)
  Product/1 -> dT_h_dt/1
  Constant1/1 -> Product/2
  Sum/1 -> Product/1
  Q_h/1 -> Sum/2
  Subsystem2/1(QV_h_e) -> Sum/3
  Subsystem1/1(QV_h_i) -> Sum/1, QV_h_i/1
  T_e/1 -> Subsystem2/1(Te)
  Th/1 -> Subsystem1/3(Th), Subsystem2/3(Th)
  Constant/1 -> Subsystem1/2(A_h_exp)
  T_i/1 -> Subsystem1/1(Ti)

== system HORTISIM/Climate/Controls/Heating Controler/Subsystem2 ==
  " Min" : Inport
  Max : Inport  Port=2
  T : Inport  Port=3
  If : If  NumInputs=3  IfExpression=u2 > u1  ElseIfExpressions=u2 < u3
  If Action Subsystem : Subsystem  TreatAsAtomicUnit=on
  If Action Subsystem1 : Subsystem  TreatAsAtomicUnit=on
  If Action Subsystem2 : Subsystem  TreatAsAtomicUnit=on
  Memory : Memory
  Merge : Merge  Inputs=3
  y : Outport
  wires:
  T/1 -> If/2
  " Min"/1 -> If/3
  Max/1 -> If/1
  If/1 -> If Action Subsystem/Action
  If/2 -> If Action Subsystem1/Action
  If/3 -> If Action Subsystem2/Action
  If Action Subsystem2/1(Out1) -> Merge/3
  If Action Subsystem1/1(Out1) -> Merge/2
  If Action Subsystem/1(Out1) -> Merge/1
  Merge/1 -> Memory/1, y/1
  Memory/1 -> If Action Subsystem2/1(In1)

== system HORTISIM/Climate/Controls/Screen Controler/Subsystem ==
  In1 : Inport
  If : If  IfExpression=u1 < 10
  If Action Subsystem : Subsystem  TreatAsAtomicUnit=on
  If Action Subsystem1 : Subsystem  TreatAsAtomicUnit=on
  Merge : Merge
  Smooth Rad : Subsystem
  Out1 : Outport
  wires:
  If Action Subsystem/1(Out1) -> Merge/1
  If/1 -> If Action Subsystem/Action
  In1/1 -> Smooth Rad/1(In1), If Action Subsystem1/1(EC)
  Merge/1 -> Out1/1
  If Action Subsystem1/1(Out1) -> Merge/2
  Smooth Rad/1(Out1) -> If/1
  If/2 -> If Action Subsystem1/Action

== system HORTISIM/Climate/Controls/Windows Controler/Subsystem ==
  Tstart : Inport
  Ti : Inport  Port=2
  Tmax : Inport  Port=3
  HRInt : Inport  Port=4
  HRStart : Inport  Port=5
  HRMax : Inport  Port=6
  Rad : Inport  Port=7
  Constant : Constant  Value=params.RadThreshold
  Hum : Saturate  UpperLimit=params.max_night  LowerLimit=0
  "Selection " : MATLAB Function  TreatAsAtomicUnit=on
  Temp : Saturate  UpperLimit=100  LowerLimit=0
  Ventilation by Hight Humidity : MATLAB Function  TreatAsAtomicUnit=on
  Ventilation by Hight Temperature1 : MATLAB Function  TreatAsAtomicUnit=on
  y : Outport
  wires:
  Constant/1 -> "Selection "/4(Rad_threshold)
  Temp/1 -> "Selection "/2(Temperature)
  HRInt/1 -> Ventilation by Hight Humidity/1(HRInt)
  Ventilation by Hight Temperature1/1(y) -> Temp/1
  HRStart/1 -> Ventilation by Hight Humidity/2(HRStart)
  Ventilation by Hight Humidity/1(y) -> Hum/1
  "Selection "/1(y) -> y/1
  Tmax/1 -> Ventilation by Hight Temperature1/3(Tmax)
  HRMax/1 -> Ventilation by Hight Humidity/3(HRMax)
  Hum/1 -> "Selection "/3(Humidity)
  Tstart/1 -> Ventilation by Hight Temperature1/1(Tstart)
  Rad/1 -> "Selection "/1(Rad)
  Ti/1 -> Ventilation by Hight Temperature1/2(Ti)
